simulink model "logic_Operator"  (R2024b)
settings: Solver=VariableStepAuto  StartTime=0.0  StopTime=10.0  RelTol=1e-3
libraries: simulink x9
settings Model: Creator=abdal  LastModifiedBy=abdal

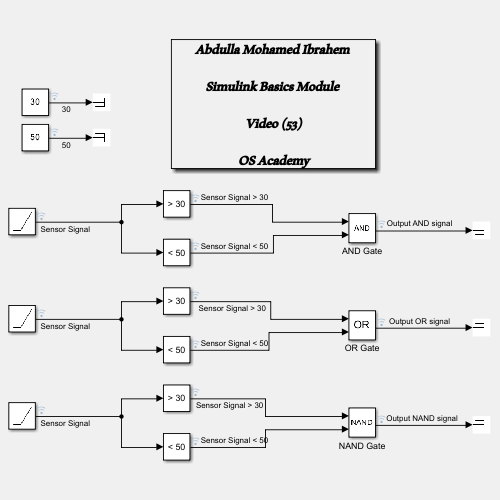
[thumbnail: Simulink's stored preview of the top-level diagram]
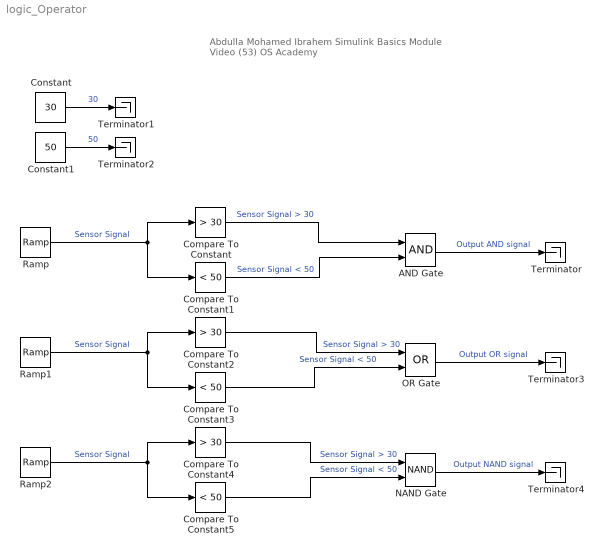
== system logic_Operator ==
  note: Abdulla Mohamed Ibrahem
      | Simulink Basics Module
      | Video (53)
      | OS Academy
  AND Gate : Logic  AllPortsSameDT=off  OutDataTypeStr=boolean
  Compare To Constant : simulink/Logic and Bit Operations/Compare To Constant  relop=>  const=30  OutDataTypeStr=boolean
  Compare To Constant1 : simulink/Logic and Bit Operations/Compare To Constant  relop=<  const=50  OutDataTypeStr=boolean
  Compare To Constant2 : simulink/Logic and Bit Operations/Compare To Constant  relop=>  const=30  OutDataTypeStr=boolean
  Compare To Constant3 : simulink/Logic and Bit Operations/Compare To Constant  relop=<  const=50  OutDataTypeStr=boolean
  Compare To Constant4 : simulink/Logic and Bit Operations/Compare To Constant  relop=>  const=30  OutDataTypeStr=boolean
  Compare To Constant5 : simulink/Logic and Bit Operations/Compare To Constant  relop=<  const=50  OutDataTypeStr=boolean
  Constant : Constant  Value=30
  Constant1 : Constant  Value=50
  NAND Gate : Logic  Operator=NAND  AllPortsSameDT=off  OutDataTypeStr=boolean
  OR Gate : Logic  Operator=OR  AllPortsSameDT=off  OutDataTypeStr=boolean
  Ramp : simulink/Sources/Ramp  slope=7  start=0  InitialOutput=0
  Ramp1 : simulink/Sources/Ramp  slope=7  start=0  InitialOutput=0
  Ramp2 : simulink/Sources/Ramp  slope=7  start=0  InitialOutput=0
  Terminator{,1..4} (5 alike) : Terminator
  wires:
  Compare To Constant/1 -> AND Gate/1  "Sensor Signal > 30"
  Compare To Constant1/1 -> AND Gate/2  "Sensor Signal < 50"
  Ramp/1 -> Compare To Constant1/1, Compare To Constant/1  "Sensor Signal"
  AND Gate/1 -> Terminator/1  "Output AND signal"
  Constant1/1 -> Terminator2/1  "50"
  Constant/1 -> Terminator1/1  "30"
  OR Gate/1 -> Terminator3/1  "Output OR signal"
  Ramp1/1 -> Compare To Constant2/1, Compare To Constant3/1  "Sensor Signal"
  Compare To Constant3/1 -> OR Gate/2  "Sensor Signal < 50"
  Compare To Constant2/1 -> OR Gate/1  "Sensor Signal > 30"
  Compare To Constant4/1 -> NAND Gate/1  "Sensor Signal > 30"
  Compare To Constant5/1 -> NAND Gate/2  "Sensor Signal < 50"
  Ramp2/1 -> Compare To Constant5/1, Compare To Constant4/1  "Sensor Signal"
  NAND Gate/1 -> Terminator4/1  "Output NAND signal"
